simulink model "basic_ref_generation"  (R2023b)
settings: Solver=VariableStepAuto  StartTime=0.0  StopTime=10.0  RelTol=1e-3
libraries: simulink x1
settings Model: Creator=bglen  LastModifiedBy=bglen

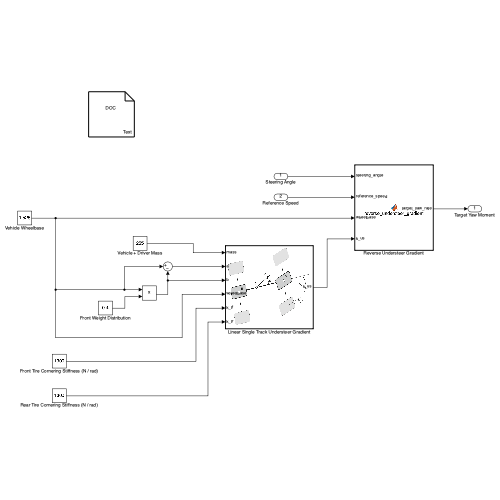
[thumbnail: Simulink's stored preview of the top-level diagram]
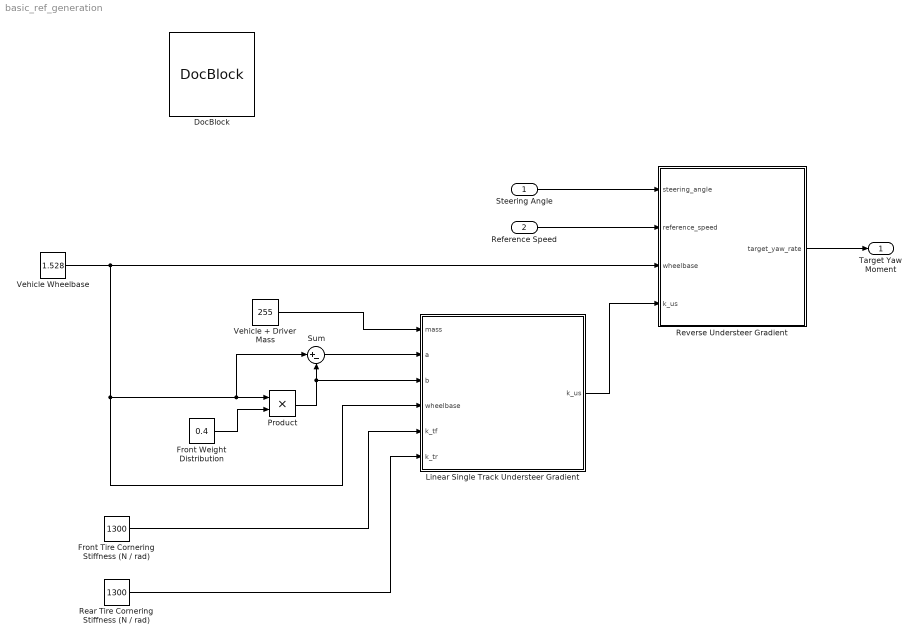
== system basic_ref_generation ==
  Steering Angle : Inport
  Reference Speed : Inport  Port=2
  DocBlock : simulink/Model-Wide Utilities/DocBlock  DocumentType=Text
      content=|
      | Basic Reference Generation
      |
      | This is the simplest form of yaw rate reference generation and also the least useful.
      | It is really only useful for lateral accelerations up to 0.4G, where tire behavior is mostly linear.
      |
      | This block provides a yaw rate linearly proportional to steering angle as:
      |
      | Y_ref = V / (l * (1 + K_us * V^2) * delta
      |
      | Where k_us is based on a steady-state linear single track model:
      |
      | k_us = (m / l^2) * (b / k_tf - a / k_tr)
      |
      | Where:
      | Y_ref: reference yaw rate
      | V: refence speed
      | l: wheelbase
      | k_us: understeer coefficient
      | delta: steering angle
      | m: total vehicle mass
      | a: CoG to front axle distance
      | b: CoG to rear axle distance
      | k_tf: front tire cornering stiffness
      | k_tr: rear tire cornering stiffness
      |
      | Vehicle Model Assumptions:
      | - Steering angle is the same on both front tires.
      | - No lateral load transfer
      | - The velocity of the vehicle’s center of gravity is considered to be constant
      | along the longitude of its trajectory.
      | - All lifting, rolling and pitching motion will be neglected.
      | - The vehicle’s mass is assumed to be concentrated at the center of gravity.
      | - The front and the rear tires will be represented as one single tire on each axle.
      | The imaginary tire contact points which the tire forces are to act upon,
      | lie along the center of the axle.
      | - The pneumatic trail and the aligning torque resulting from the slip angle of the
      | tire will be neglected.
      | - The wheel-load distribution between front and rear axle is assumed to be
      | constant.
      | - The longitudinal forces on the tires, resulting from the assumption of a constant
      | longitudinal velocity, will be neglected.
  Front Tire Cornering Stiffness (N / rad) : Constant  Value=1300
  Front Weight Distribution : Constant  Value=0.4
  Linear Single Track Understeer Gradient : MATLAB Function  TreatAsAtomicUnit=on
  Product : Product
  Rear Tire Cornering Stiffness (N / rad) : Constant  Value=1300
  Reverse Understeer Gradient : MATLAB Function  TreatAsAtomicUnit=on
  Sum : Sum  Inputs=|+-
  Vehicle + Driver Mass : Constant  Value=255
  Vehicle Wheelbase : Constant  Value=1.528
  Target Yaw Moment : Outport
  wires:
  Reverse Understeer Gradient/1(target_yaw_rate) -> Target Yaw Moment/1
  Steering Angle/1 -> Reverse Understeer Gradient/1(steering_angle)
  Reference Speed/1 -> Reverse Understeer Gradient/2(reference_speed)
  Linear Single Track Understeer Gradient/1(k_us) -> Reverse Understeer Gradient/4(k_us)
  Front Weight Distribution/1 -> Product/2
  Product/1 -> Linear Single Track Understeer Gradient/3(b), Sum/2
  Vehicle Wheelbase/1 -> Reverse Understeer Gradient/3(wheelbase), Sum/1, Product/1, Linear Single Track Understeer Gradient/4(wheelbase)
  Vehicle + Driver Mass/1 -> Linear Single Track Understeer Gradient/1(mass)
  Sum/1 -> Linear Single Track Understeer Gradient/2(a)
  Front Tire Cornering Stiffness (N / rad)/1 -> Linear Single Track Understeer Gradient/5(k_tf)
  Rear Tire Cornering Stiffness (N / rad)/1 -> Linear Single Track Understeer Gradient/6(k_tr)

== matlab function basic_ref_generation/Linear Single Track Understeer Gradient ==
  data: mass input; k_us output; a input; b input; wheelbase input; k_tf input; k_tr input
%{
Calculation of understeer coefficient given linear single track parameters

mass: Mass of vehicle and driver
a: distance from CoG to front axle
b: distance from CoG to rear axle
k_tf: front tire cornering stiffness
k_tr: rear tire cornering stiffness

Notes:
- cornering stiffness is linear
- these are steady state equations, model does not consider transient
spring and damping during transient manuevers

%}
function k_us = fcn(mass, a, b, wheelbase, k_tf, k_tr)

k_us = (mass / wheelbase^2) * (b / k_tf - a / k_tr);

== matlab function basic_ref_generation/Reverse Understeer Gradient ==
  data: steering_angle input; target_yaw_rate output; reference_speed input; wheelbase input; k_us input
%{
This function calculates the target yaw rate given the steering angle and
reference speed of a vehicle, and assumes a linear single track vehicle
model to derive understeer gradient from.

Units:
- Reference Speed: m/s
- Wheelbase: m
- Steering Angle: rad

%}

function target_yaw_rate = reverse_understeer_gradient(steering_angle, reference_speed, wheelbase, k_us)

target_yaw_rate = reference_speed / (wheelbase*(1 + k_us * reference_speed^2)) * steering_angle;
